simulink library "LineFollower"  (R2018b)
settings: Solver=VariableStepAuto  StartTime=0.0  StopTime=10.0  RelTol=1e-3
settings Model: Creator=Sjoerd  LastModifiedBy=Sjoerd

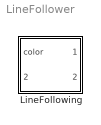
== system LineFollower ==
  "LineFollowing " : Stateflow chart  TreatAsAtomicUnit=on

== stateflow chart LineFollower/LineFollowing  ==
  state Backup
    leftMotor = -20
    rightMotor = -10
  note: Turn left
  note: Turn right
  state FollowLine
  (default) -> Backup : {maxPower = 30}
  Backup -> FollowLine : after(200,msec)
  FollowLine -> FollowLine [order 1] : [color > 70]{rightMotor = 0;leftMotor = maxPower}
  FollowLine -> FollowLine [order 4] : [color < 12]{leftMotor = -20; rightMotor = 0;}
  FollowLine -> FollowLine [order 5] : [color < homeColor-10]{leftMotor = maxPower /2 ; rightMotor = maxPower}
  FollowLine -> FollowLine [order 2] : [color > homeColor+10]{rightMotor = maxPower /2; leftMotor = maxPower}
  FollowLine -> FollowLine [order 6] : [color < homeColor]{leftMotor = maxPower - 5; rightMotor = maxPower}
  FollowLine -> FollowLine [order 7] : {leftMotor = maxPower; rightMotor = maxPower}
  FollowLine -> FollowLine [order 3] : [color > homeColor]{rightMotor = maxPower - 5; leftMotor = maxPower}
  data: maxPower local int32; color input; leftMotor output int32 size=1; rightMotor output int32 size=1; homeColor input =20
